simulink model "W04_2_turn"  (R2024b)
settings: Solver=ode4  StartTime=0.0  StopTime=80  FixedStep=0.05  RelTol=1e-3
values from neighbouring files (symbols this model uses):
  animate = 1    [W04_setup.m]
libraries: ros2lib x5
settings Model: Creator=admin  LastModifiedBy=admin

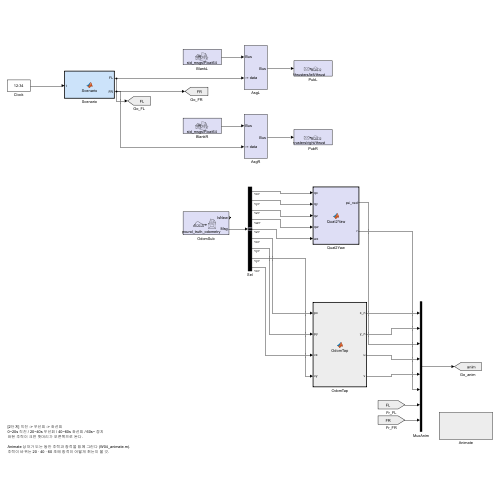
[thumbnail: Simulink's stored preview of the top-level diagram]
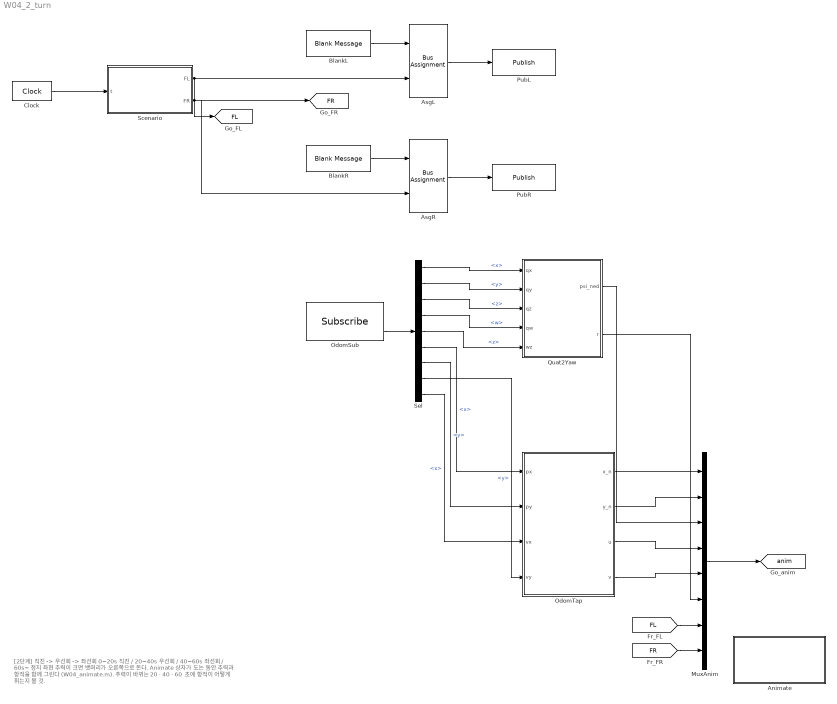
== system W04_2_turn ==
  note: [2단계] 직진 -> 우선회 -> 좌선회
      | 0~20s 직진 / 20~40s 우선회 / 40~60s 좌선회 / 60s~ 정지
      | 좌현 추력이 크면 뱃머리가 오른쪽으로 돈다.
      |
      | Animate 상자가 도는 동안 추력과 항적을 함께 그린다 (W04_animate.m).
      | 추력이 바뀌는 20 · 40 · 60 초에 항적이 어떻게 휘는지 볼 것.
  Animate : Subsystem
  AsgL : BusAssignment  AssignedSignals=data
  AsgR : BusAssignment  AssignedSignals=data
  BlankL : ros2lib/Blank Message  messageClass=Message  entityType=std_msgs/Float64  messageType=std_msgs/Float64  SampleTime=0.05
  BlankR : ros2lib/Blank Message  messageClass=Message  entityType=std_msgs/Float64  messageType=std_msgs/Float64  SampleTime=0.05
  Clock : DigitalClock  SampleTime=0.05
  MuxAnim : Mux  Inputs=8
  OdomSub : ros2lib/Subscribe  topicSource=Specify your own  topic=/wamv/sensors/position/ground_truth_odometry  messageType=nav_msgs/Odometry  sampleTime=0.05  QOSHistory=Keep last  QOSDepth=1  QOSReliability=Reliable  QOSDurability=Volatile  QOSDeadline=Inf  QOSLifespan=Inf  QOSLiveliness=Automatic  QOSLeaseDuration=Inf  QOSAvoidROSNamespaceConventions=off
  OdomTap : MATLAB Function  TreatAsAtomicUnit=on
  PubL : ros2lib/Publish  topicSource=Specify your own  topic=/wamv/thrusters/left/thrust  messageType=std_msgs/Float64  QOSHistory=Keep last  QOSDepth=1  QOSReliability=Reliable  QOSDurability=Volatile  QOSDeadline=Inf  QOSLifespan=Inf  QOSLiveliness=Automatic  QOSLeaseDuration=Inf  QOSAvoidROSNamespaceConventions=off
  PubR : ros2lib/Publish  topicSource=Specify your own  topic=/wamv/thrusters/right/thrust  messageType=std_msgs/Float64  QOSHistory=Keep last  QOSDepth=1  QOSReliability=Reliable  QOSDurability=Volatile  QOSDeadline=Inf  QOSLifespan=Inf  QOSLiveliness=Automatic  QOSLeaseDuration=Inf  QOSAvoidROSNamespaceConventions=off
  Quat2Yaw : MATLAB Function  TreatAsAtomicUnit=on
  Scenario : MATLAB Function  TreatAsAtomicUnit=on
  Sel : BusSelector  OutputSignals=pose.pose.orientation.x,pose.pose.orientation.y,pose.pose.orientation.z,pose.pose.orientation.w,twist.twist.angular.z,pose.pose.position.x,pose.pose.position.y,twist.twist.linear.y,twist.twist.linear.x
  tag scope: FL=global, FR=global, anim=global
  wires:
  BlankL/1 -> AsgL/1
  AsgL/1 -> PubL/1
  BlankR/1 -> AsgR/1
  AsgR/1 -> PubR/1
  Clock/1 -> Scenario/1(t)
  Scenario/1(FL) -> AsgL/2, [FL]
  OdomSub/2 -> Sel/1
  Sel/1 -> Quat2Yaw/1(qx)  "<x>"
  Sel/2 -> Quat2Yaw/2(qy)  "<y>"
  Sel/3 -> Quat2Yaw/3(qz)  "<z>"
  Sel/4 -> Quat2Yaw/4(qw)  "<w>"
  Sel/5 -> Quat2Yaw/5(wz)  "<z>"
  Sel/6 -> OdomTap/1(px)  "<x>"
  Sel/7 -> OdomTap/2(py)  "<y>"
  Sel/9 -> OdomTap/3(vx)  "<x>"
  Sel/8 -> OdomTap/4(vy)  "<y>"
  OdomTap/1(x_n) -> MuxAnim/1
  OdomTap/2(y_n) -> MuxAnim/2
  OdomTap/3(u) -> MuxAnim/4
  OdomTap/4(v) -> MuxAnim/5
  Quat2Yaw/2(r) -> MuxAnim/6
  [FL] -> MuxAnim/7
  [FR] -> MuxAnim/8
  MuxAnim/1 -> [anim]
  Quat2Yaw/1(psi_ned) -> MuxAnim/3
  Scenario/2(FR) -> AsgR/2, [FR]

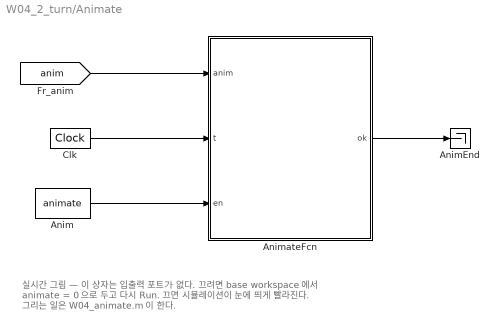
== system W04_2_turn/Animate ==
  note: 실시간 그림 — 이 상자는 입출력 포트가 없다.
      | 끄려면 base workspace 에서  animate = 0  으로 두고 다시 Run.
      | 끄면 시뮬레이션이 눈에 띄게 빨라진다.
      | 그리는 일은 W04_animate.m 이 한다.
  Anim : Constant  Value=animate
  AnimEnd : Terminator
  AnimateFcn : MATLAB Function  TreatAsAtomicUnit=on
  Clk : DigitalClock  SampleTime=0.05
  wires:
  [anim] -> AnimateFcn/1(anim)
  Clk/1 -> AnimateFcn/2(t)
  Anim/1 -> AnimateFcn/3(en)
  AnimateFcn/1(ok) -> AnimEnd/1

== matlab function W04_2_turn/Quat2Yaw ==
  data: qx input; psi_ned output; qy input; qz input; qw input; wz input; r output
function [psi_ned, r] = Quat2Yaw(qx, qy, qz, qw, wz)
%#codegen
% ROS quaternion (ENU body) -> NED heading [rad] and yaw rate [rad/s]
yaw_enu = atan2(2*(qw*qz + qx*qy), 1 - 2*(qy*qy + qz*qz));
psi = pi/2 - yaw_enu;
psi_ned = atan2(sin(psi), cos(psi));   % wrap to [-pi, pi]

% psi_ned = pi/2 - yaw_enu  ->  d(psi_ned)/dt = -d(yaw_enu)/dt.
% ENU is z-up and NED is z-down, so the turn direction flips.
r = -wz;

== matlab function W04_2_turn/Scenario ==
  data: t input; FL output; FR output
function [FL, FR] = Scenario(t)
%#codegen
% Time-based thrust scenario [N]
if t < 20
    FL = 200;  FR = 200;   % go straight
elseif t < 40
    FL = 300;  FR =  50;   % turn starboard (right)
elseif t < 60
    FL =  50;  FR = 300;   % turn port (left)
else
    FL = 0;    FR = 0;     % stop
end

== matlab function W04_2_turn/OdomTap ==
  data: px input; x_n output; py input; vx input; vy input; y_n output; u output; v output
function [x_n, y_n, u, v] = OdomTap(px, py, vx, vy)
%#codegen
% Ground truth odometry -> the numbers the live plot draws.
% Display only: nothing here feeds the controller.
x_n = py;      % ENU y is north
y_n = px;      % ENU x is east
u   =  vx;     % surge is the same in FLU and NED body axes
v   = -vy;     % FLU +y is port, NED +y is starboard

== matlab function W04_2_turn/Animate/AnimateFcn ==
  data: anim input; ok output; t input; en input
function ok = AnimateFcn(anim, t, en)
%#codegen
% 실시간 그림. MATLAB Function 블록은 그림을 그리지 못하므로 그리는 함수를
% extrinsic 으로 선언한다 — 코드를 만들지 않고 평범한 MATLAB 을 부른다.
% en = base workspace 의 animate (0 이면 그리지 않는다).
%
% anim 은 Mux 로 묶어 온 여덟 신호다 (빌더의 animBundle 과 같은 순서).
%   1 x_n   2 y_n   3 psi   4 u   5 v   6 r   7 FL   8 FR
coder.extrinsic('W04_animate');
ok = 1;
if en > 0.5
    W04_animate(anim(1), anim(2), anim(3), anim(4), anim(5), anim(6), anim(7), anim(8), NaN, NaN, t);
end
